simulink model "zbiornik_test_linmod"  (R2021b)
settings: Solver=ode45  StartTime=0.0  StopTime=inf  FixedStep=1e-3  MaxStep=0.2  RelTol=1e-3  EnableMultiTasking=on
settings Model: Creator=Stefan  LastModifiedBy=adria
settings SolverCC: AlgebraicLoopSolver=TrustRegion
settings DataIOCC: LimitDataPoints=on  SaveFormat=Array  SignalLoggingSaveFormat=ModelDataLogs  ReturnWorkspaceOutputs=off  SignalLoggingName=sigsOut
settings OptimizationCC: BooleanDataType=off  ExpressionDepthLimit=2147483647  InitFltsAndDblsToZero=on  LifeSpan=inf
settings DebuggingCC: SaveWithParameterizedLinksMsg=none  UnderspecifiedInitializationDetection=Classic  MergeDetectMultiDrivingBlocksExec=none  SignalResolutionControl=TryResolveAllWithWarning  MultiTaskDSMMsg=warning  MultiTaskCondExecSysMsg=none  FcnCallInpInsideContextMsg=warning  StateNameClashWarn=warning  SFUnexpectedBacktrackingDiag=warning  SFNoUnconditionalDefaultTransitionDiag=warning  SFExecutionAtInitializationDiag=none  SFMachineParentedDataDiag=warning  ArithmeticOperatorsInVariantConditions=warning
settings HardwareCC: ProdBitPerPointer=32  ProdBitPerSizeT=32  ProdBitPerPtrDiffT=32  ProdLargestAtomicFloat=None  ProdIntDivRoundTo=Undefined  ProdEndianess=Unspecified  ProdWordSize=32  ProdHWDeviceType=32-bit Generic  TargetUnknown=on
settings ModelReferenceCC: PropagateSignalLabelsOutOfModel=off
settings SFSimCC: SimUseLocalCustomCode=off  CustomCodeUndefinedFunction=UseInterfaceOnly
settings RTWCC: RTWUseLocalCustomCode=off
settings CodeAppCC: StateflowObjectComments=on
settings GRTTargetCC: TargetFcnLib=ansi_tfl_tmw.mat  TargetLangStandard=C89/C90 (ANSI)  CombineOutputUpdateFcns=off  GRTInterface=on
settings ConfigComp: CovMetricSettings=dw  CovSaveCumulativeToWorkspaceVar=on  CovSaveSingleToWorkspaceVar=on  CovExternalEMLEnable=off

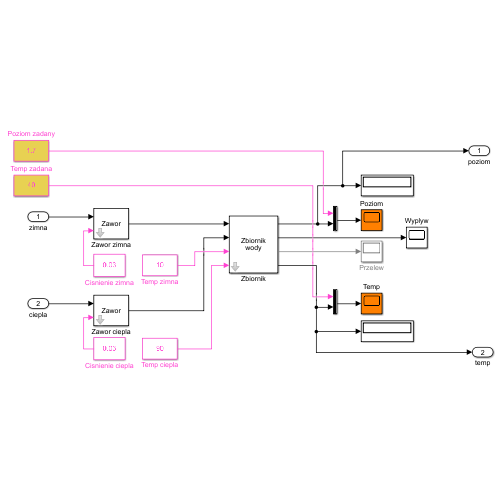
[thumbnail: Simulink's stored preview of the top-level diagram]
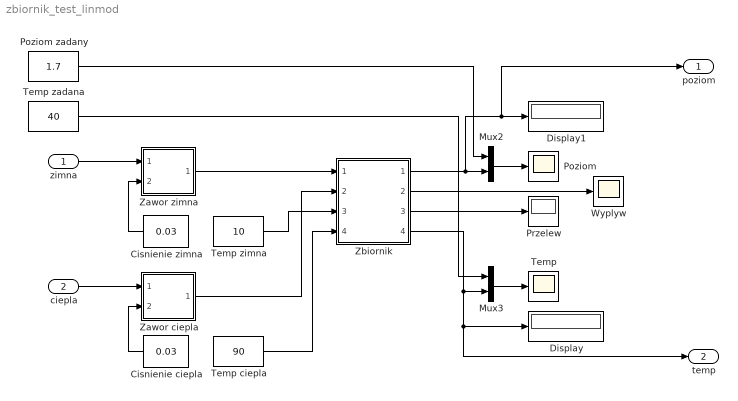
== system zbiornik_test_linmod ==
  zimna : Inport
  ciepla : Inport  Port=2
  Cisnienie ciepla : Constant  Value=0.03
  Cisnienie zimna : Constant  Value=0.03
  Display : Display
  Display1 : Display
  Mux2 : Mux  Inputs=2
  Mux3 : Mux  Inputs=2
  Poziom : Scope
  Poziom zadany : Constant  Value=1.7
  Przelew : Display
  Temp : Scope
  Temp ciepla : Constant  Value=90
  Temp zadana : Constant  Value=40
  Temp zimna : Constant  Value=10
  Wyplyw : Scope
  Zawor ciepla : Subsystem  mask(Valve){InitialPosition=0}
      mask prompts: InitialPosition "Initial position [0=closed 1=open]:"
      mask help: Valve
      mask Display: disp('Zawor')
  Zawor zimna : Subsystem  mask(Valve){InitialPosition=0}
      mask prompts: InitialPosition "Initial position [0=closed 1=open]:"
      mask help: Valve
      mask Display: disp('Zawor')
  Zbiornik : Subsystem  mask(Zbiornik wody){ht=2, area=5, outletArea=0.005, overflowLimit=0, initialHt=0.5}
      mask prompts: ht "Wysokosc zbiornika (m):"; area "Przekroj zbiornika (m^2):"; outletArea "Przekroj wyplywu (m^2):"; overflowLimit "Pozycja czujnika alarmu(m):"; initialHt "Poziom poczatkowy (m):"
      mask help: Zbiornik wody ze swobodnym wyplywem
      mask Display: disp('Zbiornik\nwody')
  poziom : Outport
  temp : Outport  Port=2
  wires:
  Zbiornik/2(flow out) -> Wyplyw/1
  Cisnienie zimna/1 -> Zawor zimna/2(source flow)
  Zbiornik/1(water level) -> poziom/1, Display1/1, Mux2/2
  Zbiornik/3(overflow flag) -> Przelew/1
  Mux2/1 -> Poziom/1
  Poziom zadany/1 -> Mux2/1
  Cisnienie ciepla/1 -> Zawor ciepla/2(source flow)
  Zawor zimna/1(out flow) -> Zbiornik/1(flow_cold_in)
  Zawor ciepla/1(out flow) -> Zbiornik/2(flow_hot_in)
  Temp zimna/1 -> Zbiornik/3(temp_cold_in)
  Temp ciepla/1 -> Zbiornik/4(temp_hot_in)
  Mux3/1 -> Temp/1
  Temp zadana/1 -> Mux3/1
  Zbiornik/4(temp_out) -> temp/1, Display/1, Mux3/2
  zimna/1 -> Zawor zimna/1(control)
  ciepla/1 -> Zawor ciepla/1(control)

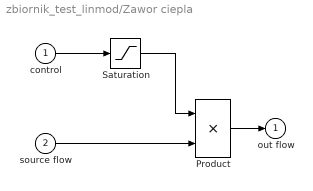
== system zbiornik_test_linmod/Zawor ciepla ==
  control : Inport
  source flow : Inport  Port=2
  Product : Product  InputSameDT=on  SaturateOnIntegerOverflow=on  OutDataTypeStr=Inherit: Same as first input
  Saturation : Saturate  UpperLimit=1  LowerLimit=0
  out flow : Outport  InitialOutput=0  VectorParamsAs1DForOutWhenUnconnected=off
  wires:
  source flow/1 -> Product/2
  Product/1 -> out flow/1
  control/1 -> Saturation/1
  Saturation/1 -> Product/1

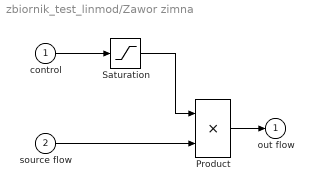
== system zbiornik_test_linmod/Zawor zimna ==
  control : Inport
  source flow : Inport  Port=2
  Product : Product  InputSameDT=on  SaturateOnIntegerOverflow=on  OutDataTypeStr=Inherit: Same as first input
  Saturation : Saturate  UpperLimit=1  LowerLimit=0
  out flow : Outport  InitialOutput=0  VectorParamsAs1DForOutWhenUnconnected=off
  wires:
  source flow/1 -> Product/2
  Product/1 -> out flow/1
  control/1 -> Saturation/1
  Saturation/1 -> Product/1

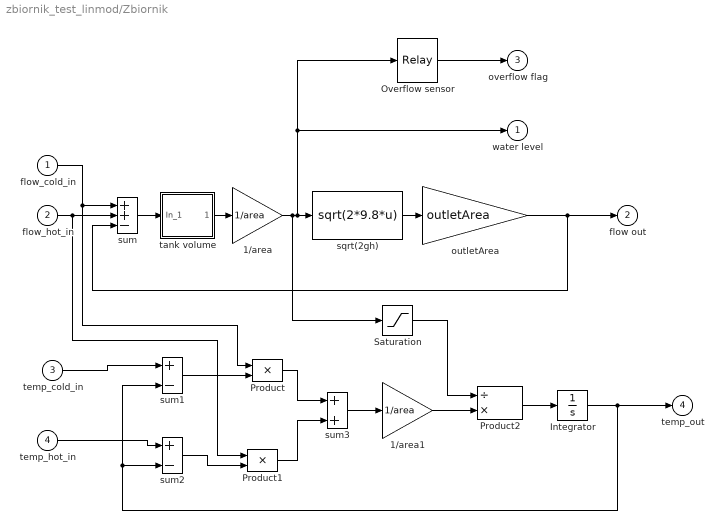
== system zbiornik_test_linmod/Zbiornik ==
  flow_cold_in : Inport
  flow_hot_in : Inport  Port=2
  temp_cold_in : Inport  Port=3
  temp_hot_in : Inport  Port=4
  1/area : Gain  Gain=1/area  SaturateOnIntegerOverflow=on  OutDataTypeStr=Inherit: Same as input  ParamDataTypeStr=Inherit: Same as input
  1/area1 : Gain  Gain=1/area  SaturateOnIntegerOverflow=on  OutDataTypeStr=Inherit: Same as input  ParamDataTypeStr=Inherit: Same as input
  Integrator : Integrator  InitialCondition=40
  Overflow sensor : Relay  OnSwitchValue=ht - overflowLimit  OffSwitchValue=ht - overflowLimit
  Product : Product  SaturateOnIntegerOverflow=on  OutDataTypeStr=Inherit: Same as first input
  Product1 : Product  SaturateOnIntegerOverflow=on  OutDataTypeStr=Inherit: Same as first input
  Product2 : Product  Inputs=/*  SaturateOnIntegerOverflow=on  OutDataTypeStr=Inherit: Same as first input
  Saturation : Saturate  UpperLimit=ht  LowerLimit=0.01
  outletArea : Gain  Gain=outletArea  SaturateOnIntegerOverflow=on  OutDataTypeStr=Inherit: Same as input  ParamDataTypeStr=Inherit: Same as input
  sqrt(2gh) : Fcn  Expr=sqrt(2*9.8*u)
  sum : Sum  Inputs=++-  InputSameDT=on  SaturateOnIntegerOverflow=on  OutDataTypeStr=Inherit: Same as first input
  sum1 : Sum  Inputs=+-  InputSameDT=on  SaturateOnIntegerOverflow=on  OutDataTypeStr=Inherit: Same as first input
  sum2 : Sum  Inputs=+-  InputSameDT=on  SaturateOnIntegerOverflow=on  OutDataTypeStr=Inherit: Same as first input
  sum3 : Sum  InputSameDT=on  SaturateOnIntegerOverflow=on  OutDataTypeStr=Inherit: Same as first input
  tank volume : Subsystem  mask(Limited integrator.){lb=0, ub=ht * area, xi=initialHt * area}
      mask prompts: lb "Lower bound:"; ub "Upper bound:"; xi "Initial condition"
      mask help: Limited integrator
      mask Help: Implements a limited integrator with \nan expression of the form:\n\nif(x<=lb and u<0) or (x>=ub and u>0)\n\txdot=0\nelse\n\txdot=u.
      mask Display: plot(-1,-0.2,3.5,1.2,[0.05,1,2,2.9],[0,0,1,1]);disp(' 1/s    ')
  water level : Outport  InitialOutput=0  VectorParamsAs1DForOutWhenUnconnected=off
  flow out : Outport  Port=2  InitialOutput=0  VectorParamsAs1DForOutWhenUnconnected=off
  overflow flag : Outport  Port=3  InitialOutput=0  VectorParamsAs1DForOutWhenUnconnected=off
  temp_out : Outport  Port=4  InitialOutput=0  VectorParamsAs1DForOutWhenUnconnected=off
  wires:
  outletArea/1 -> flow out/1, sum/3
  sqrt(2gh)/1 -> outletArea/1
  1/area/1 -> Overflow sensor/1, water level/1, sqrt(2gh)/1, Saturation/1
  tank volume/1(Out_1) -> 1/area/1
  Overflow sensor/1 -> overflow flag/1
  sum/1 -> tank volume/1(In_1)
  flow_cold_in/1 -> sum/1, Product/1
  flow_hot_in/1 -> sum/2, Product1/1
  temp_cold_in/1 -> sum1/1
  temp_hot_in/1 -> sum2/1
  sum1/1 -> Product/2
  sum2/1 -> Product1/2
  Product/1 -> sum3/1
  Product1/1 -> sum3/2
  sum3/1 -> 1/area1/1
  1/area1/1 -> Product2/2
  Product2/1 -> Integrator/1
  Integrator/1 -> temp_out/1, sum2/2, sum1/2
  Saturation/1 -> Product2/1

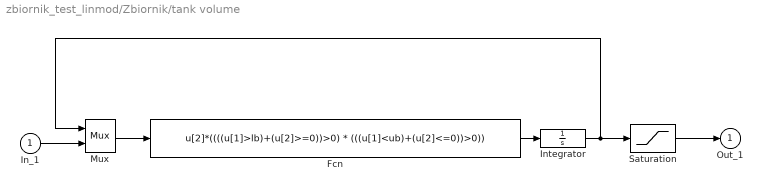
== system zbiornik_test_linmod/Zbiornik/tank volume ==
  In_1 : Inport
  Fcn : Fcn  Expr=u[2]*((((u[1]>lb)+(u[2]>=0))>0) * (((u[1]<ub)+(u[2]<=0))>0))
  Integrator : Integrator  InitialCondition=xi
  Mux : Mux  Inputs=2
  Saturation : Saturate  UpperLimit=ub  LowerLimit=lb
  Out_1 : Outport  InitialOutput=0  VectorParamsAs1DForOutWhenUnconnected=off
  wires:
  Integrator/1 -> Saturation/1, Mux/1
  Fcn/1 -> Integrator/1
  Mux/1 -> Fcn/1
  In_1/1 -> Mux/2
  Saturation/1 -> Out_1/1
